simulink model "dataset_generator"  (R2021a)
settings: Solver=VariableStepAuto  StartTime=0.0  StopTime=Tf  RelTol=1e-3
libraries: vrlib x1, dspvision x1, visionsinks x1
settings Model: Creator=tkikawad  LastModifiedBy=tkikawad
settings SolverCC: AlgebraicLoopSolver=TrustRegion
settings DebuggingCC: SFMachineParentedDataDiag=warning

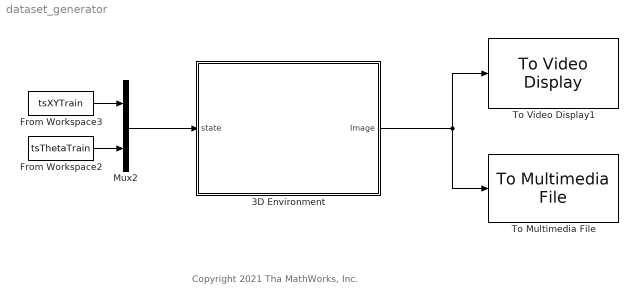
== system dataset_generator ==
  note: Copyright 2021 Tha MathWorks, Inc.
  3D Environment : Subsystem  mask{world=World1, z=0}
      mask prompts: world "Select World:"
      mask init:
      | switch world
      |   case 1
      |     z = 0;
      |     imgfile =  'course.png';
      |   case 2
      |     z = 10;
      |     imgfile =  'course_circle.png';
      |   case 3
      |     z = 20;
      |     imgfile =  'course_curve.png';
      |   otherwise
      |     imgfile =  'course.png';
      | end
      | assignin('base','world',world)
      mask TypeOptions world: World1 | World2 | World3
      mask DialogControl DescGroupVar Prompt: 3D Environment
      mask DialogControl DescTextVar Prompt: 3D environment using Simulink 3D Animation.
      mask Display:
      | image(imgfile,[0.15 0.15 0.7 0.7]);
      | text(0.5, 0.1, "World" + world,...
      |     'horizontalAlignment', 'center',...
      |     'verticalAlignment', 'top');
  From Workspace2 : FromWorkspace  VariableName=tsThetaTrain  SampleTime=0.1
  From Workspace3 : FromWorkspace  VariableName=tsXYTrain  SampleTime=0.1
  Mux2 : Mux  Inputs=2
  To Multimedia File : dspvision/To Multimedia File  outputFilename=robotTrain.avi  streamSelection=Video only  videoCompressor=None (uncompressed)  audioCompressor=None (uncompressed)  imagePorts=One multidimensional signal  fileType=AVI  audioDatatype=Determine from input data type  fourcc=RGB  videoQuality=75  mj2000CompFactor=10
  To Video Display1 : visionsinks/To Video Display  windowSizeMode=Normal  openAtMdlStart=on  fullScreen=off  videoWindowX=641  videoWindowY=87  saveWindowSize=off  videoWindowWidth=482  videoWindowHeight=301  inputColorFormat=RGB  inputType=Obsolete  imagePorts=One multidimensional signal  OutputDevice=On-screen video monitor  dataOrg=Column-major  isWindowOpen=off
  wires:
  From Workspace2/1 -> Mux2/2
  From Workspace3/1 -> Mux2/1
  Mux2/1 -> 3D Environment/1(state)
  3D Environment/1(Image) -> To Multimedia File/1, To Video Display1/1

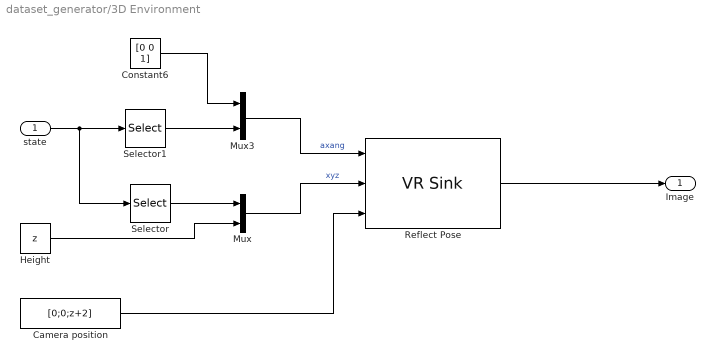
== system dataset_generator/3D Environment ==
  state : Inport
  Camera position : Constant  Value=[0;0;z+2]
  Constant6 : Constant  Value=[0 0 1]
  Height : Constant  Value=z
  Mux : Mux  Inputs=2
  Mux3 : Mux  Inputs=2
  Reflect Pose : vrlib/VR Sink  InstantiateOnLoad=on  SampleTime=0.1  ViewEnable=on  RemoteChange=off  RemoteView=off  FieldsWritten=robot.rotation.4.1.1.double#robot.translation.3.1.1.double#worldCamera.position.3.1.1.double  WorldFileName=robotTrainWorld.wrl  AutoView=on  VideoDimensions=[180,320]  AllowVariableSize=off  FigureProperties="{'Position', 'Name', 'Viewpoint', 'CameraBound', 'CameraDirection', 'CameraPosition', 'CameraUpVector', 'ZoomFactor', 'Antialiasing', 'Headlight', 'Lighting', 'NavPanel', 'Sound', 'StatusBar', 'Stereo3D', 'Stereo3DCameraOffset', 'Stereo3DHIT', 'ToolBar', 'Textures', 'Transparency', 'Triad', 'Wireframe', 'NavZones', 'NavMode', 'NavSpeed', 'CaptureFileFormat', 'CaptureFileName', 'Record2DCompressMethod', 'Record2DCompressQuality', 'Record2D', 'Record2DFileName', 'Record2DFPS'; [5.0000000000000000e+00   9.2000000000000000e+01   5.7600000000000000e+02   3.5000000000000000e+02], '', '_untitled_2', 'on', [0.0000000000000000e+00   0.0000000000000000e+00  -1.0000000000000000e+00], [0.0000000000000000e+00   0.0000000000000000e+00   0.0000000000000000e+00], [0.0000000000000000e+00   1.0000000000000000e+00   0.0000000000000000e+00], [1.0000000000000000e+00], 'off', 'on', 'on', 'halfbar', 'on', 'on', 'off', [1.0000000149011612e-01], [0.0000000000000000e+00], 'on', 'on', 'on', 'none', 'off', 'off', 'fly', 'normal', 'tif', '%f_anim_%n.tif', 'auto', [7.5000000000000000e+01], 'off', '%f_anim_%n.avi', 'auto'; [5.8600000000000000e+02   6.0000000000000000e+01   3.2000000000000000e+02   1.8000000000000000e+02], '', '_untitled_1', 'on', [0.0000000000000000e+00   0.0000000000000000e+00  -1.0000000000000000e+00], [0.0000000000000000e+00   0.0000000000000000e+00   0.0000000000000000e+00], [0.0000000000000000e+00   1.0000000000000000e+00   0.0000000000000000e+00], [1.0000000000000000e+00], 'on', 'on', 'on', 'none', 'on', 'off', 'off', [1.0000000149011612e-01], [0.0000000000000000e+00], 'off', 'on', 'on', 'none', 'off', 'off', 'fly', 'normal', 'tif', '%f_anim_%n.tif', 'auto', [7.5000000000000000e+01], 'off', '***video***', 'auto'}"
  Selector : Selector  InputPortWidth=3  IndexOptions=Index vector (dialog)  Indices=[1 2]  OutputSizes=1
  Selector1 : Selector  InputPortWidth=3  IndexOptions=Index vector (dialog)  Indices=3  OutputSizes=1
  Image : Outport
  wires:
  Reflect Pose/1 -> Image/1
  Height/1 -> Mux/2
  Mux/1 -> Reflect Pose/2  "xyz"
  Constant6/1 -> Mux3/1
  state/1 -> Selector1/1, Selector/1
  Mux3/1 -> Reflect Pose/1  "axang"
  Selector1/1 -> Mux3/2
  Camera position/1 -> Reflect Pose/3
  Selector/1 -> Mux/1
